simulink model "Simulation"  (R2019b)
settings: Solver=ode1  StartTime=0.0  StopTime=50  FixedStep=0.002  RelTol=1e-3  EnableMultiTasking=on
values from neighbouring files (symbols this model uses):
  Co = 0.1285    [Setup_sim.m]
  Dp = 0.024*0    (= 0)    [Setup_sim.m]
  Dr = 0.0690    (= 0.069)    [Setup_sim.m]
  g = 0.981    [Setup_sim.m]
  init_condi = pi/180*[5, 5, 0, 0]    [Setup_sim.m]
  Jp = 0.0012    [Setup_sim.m]    (also in parameters.mat)
  Jr = 0.0083    [Setup_sim.m]    (also in parameters.mat = 0.0038)
  K_AMP = 1    [Setup_sim.m]
  K_CT = lqr(Ai,Bi,Qx,Qu)    [Setup_sim.m]
  Lp = 0.3111    [Setup_sim.m]    (also in parameters.mat = 0.337)
  Lr = 0.1270    (= 0.127)    [Setup_sim.m]    (also in parameters.mat)
  Mp = 0.1270    (= 0.127)    [Setup_sim.m]
  sysc = ss(A,B,C,D)    [Setup_sim.m]
  VMAX_DAC = 10    [Setup_sim.m]
undefined symbols (not defined in the file or in its folder): DiscIntNeverNeededParam, L_CT, VMAX_AMP
libraries: simulink_extras x7
settings Model: ExtModeTrigDuration=10000  Creator=MLevis  LastModifiedBy=albin
settings SolverCC: PositivePriorityOrder=on
settings DataIOCC: LimitDataPoints=on  SaveFormat=Array  SignalLoggingSaveFormat=ModelDataLogs  ReturnWorkspaceOutputs=off
settings OptimizationCC: BooleanDataType=off  OptimizeBlockIOStorage=off  BufferReuse=off  GlobalBufferReuse=off  ExpressionFolding=off  ExpressionDepthLimit=2147483647  LocalBlockOutputs=off  InitFltsAndDblsToZero=on  LifeSpan=inf  OptimizeDataStoreBuffers=off  BusAssignmentInplaceUpdate=off
settings DebuggingCC: SaveWithParameterizedLinksMsg=none  UnderspecifiedInitializationDetection=Classic  MergeDetectMultiDrivingBlocksExec=none  SignalResolutionControl=TryResolveAllWithWarning  MultiTaskDSMMsg=warning  MultiTaskCondExecSysMsg=none  FcnCallInpInsideContextMsg=warning  StateNameClashWarn=warning  SFUnexpectedBacktrackingDiag=warning  SFNoUnconditionalDefaultTransitionDiag=warning  ArithmeticOperatorsInVariantConditions=warning
settings HardwareCC: ProdBitPerPointer=32  ProdBitPerSizeT=32  ProdBitPerPtrDiffT=32  ProdLargestAtomicFloat=None  ProdIntDivRoundTo=Undefined  ProdEndianess=Unspecified  ProdWordSize=32  ProdHWDeviceType=32-bit Generic  TargetHWDeviceType=32-bit Generic
settings ModelReferenceCC: PropagateSignalLabelsOutOfModel=off
settings SFSimCC: SimUseLocalCustomCode=off  CustomCodeUndefinedFunction=UseInterfaceOnly
settings RTWCC: Description=Quarc Win32 Target  SystemTargetFile=quarc_windows.tlc  TemplateMakefile=quarc_default_tmf  RTWUseLocalCustomCode=off
settings CodeAppCC: StateflowObjectComments=on
settings STFCustomTargetCC: TargetFcnLib=ansi_tfl_tmw.mat  TargetPreCompLibLocation=C:\PROGRA~3\QUARC\lib\2015a\windows\release  GeneratePreprocessorConditionals=Disable all  CPPClassGenCompliant=on  GRTInterface=on  SystemTargetFile=quarc_windows.tlc
settings GRTTargetCC: TargetFcnLib=ansi_tfl_tmw.mat  TargetPreCompLibLocation=C:\PROGRA~3\QUARC\lib\2015a\windows\release  TargetLangStandard=C89/C90 (ANSI)  ParMdlRefBuildCompliant=off  CompOptLevelCompliant=off  ConcurrentExecutionCompliant=off  GeneratePreprocessorConditionals=Disable all  CombineOutputUpdateFcns=off  MatFileLogging=off  GRTInterface=on  UseToolchainInfoCompliant=off  ExtMode=on  ExtModeMexFile=quarc_comm
settings ConfigComp: CovMetricSettings=dw  CovHtmlReporting=on  CovSaveCumulativeToWorkspaceVar=on  CovSaveSingleToWorkspaceVar=on  CovExternalEMLEnable=off

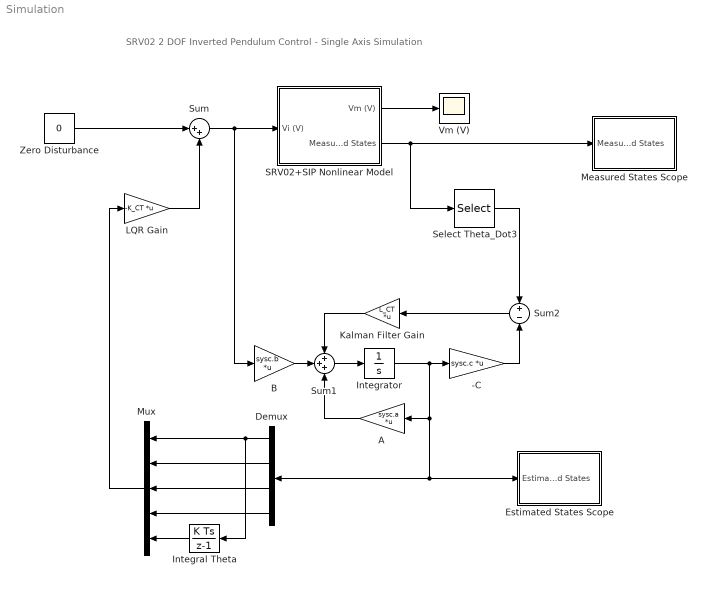
== system Simulation ==
  note: SRV02 2 DOF Inverted Pendulum Control - Single Axis Simulation
  -C : Gain  Gain=sysc.c  Multiplication=Matrix(K*u)
  A : Gain  Gain=sysc.a  Multiplication=Matrix(K*u)
  B : Gain  Gain=sysc.b  Multiplication=Matrix(K*u)
  Demux : Demux
  Estimated States Scope : Subsystem
  Integral Theta : DiscreteIntegrator  SampleTime=0.002  ICPrevOutput=DiscIntNeverNeededParam  ICPrevScaledInput=DiscIntNeverNeededParam
  Integrator : Integrator
  Kalman Filter Gain : Gain  Gain=L_CT  Multiplication=Matrix(K*u)
  LQR Gain : Gain  Gain=-K_CT  Multiplication=Matrix(K*u)  SaturateOnIntegerOverflow=on  OutDataTypeStr=Inherit: Same as input  ParamDataTypeStr=Inherit: Same as input
  Measured States Scope : Subsystem
  Mux : Mux  Inputs=5
  SRV02+SIP Nonlinear Model : Subsystem
  Select Theta_Dot3 : Selector  InputPortWidth=3  IndexOptions=Index vector (dialog)  Indices=[1 2]  OutputSizes=1
  Sum : Sum  Inputs=|++
  Sum1 : Sum  Inputs=+++
  Sum2 : Sum  Inputs=+|-
  Vm (V) : Scope
  Zero Disturbance : Constant  Value=0
  wires:
  LQR Gain/1 -> Sum/2
  B/1 -> Sum1/2
  Sum1/1 -> Integrator/1
  Integrator/1 -> Demux/1, Estimated States Scope/1(Estimated States), A/1, -C/1
  -C/1 -> Sum2/2
  Sum2/1 -> Kalman Filter Gain/1
  Kalman Filter Gain/1 -> Sum1/1
  A/1 -> Sum1/3
  Sum/1 -> SRV02+SIP Nonlinear Model/1(Vi (V)), B/1
  SRV02+SIP Nonlinear Model/2(Measured States) -> Measured States Scope/1(Measured States), Select Theta_Dot3/1
  SRV02+SIP Nonlinear Model/1(Vm (V)) -> Vm (V)/1
  Zero Disturbance/1 -> Sum/1
  Select Theta_Dot3/1 -> Sum2/1
  Demux/1 -> Integral Theta/1, Mux/1
  Demux/2 -> Mux/2
  Demux/3 -> Mux/3
  Demux/4 -> Mux/4
  Mux/1 -> LQR Gain/1
  Integral Theta/1 -> Mux/5

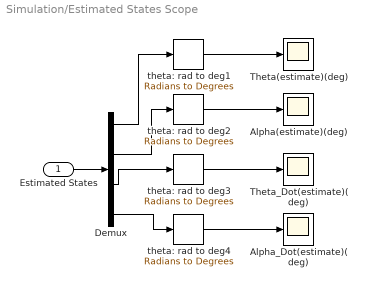
== system Simulation/Estimated States Scope ==
  Estimated States : Inport
  Alpha(estimate)(deg) : Scope
  Alpha_Dot(estimate)(deg) : Scope
  Demux : Demux
  Theta(estimate)(deg) : Scope
  Theta_Dot(estimate)(deg) : Scope
  theta: rad to deg{1..4} (4 alike) : simulink_extras/Transformations/Radians to Degrees
  wires:
  Demux/1 -> theta: rad to deg1/1
  theta: rad to deg1/1 -> Theta(estimate)(deg)/1
  theta: rad to deg2/1 -> Alpha(estimate)(deg)/1
  Demux/2 -> theta: rad to deg2/1
  theta: rad to deg3/1 -> Theta_Dot(estimate)(deg)/1
  Demux/3 -> theta: rad to deg3/1
  theta: rad to deg4/1 -> Alpha_Dot(estimate)(deg)/1
  Demux/4 -> theta: rad to deg4/1
  Estimated States/1 -> Demux/1

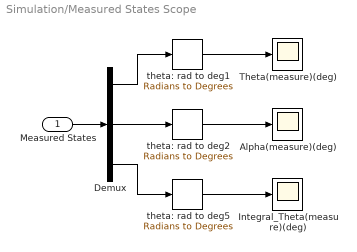
== system Simulation/Measured States Scope ==
  Measured States : Inport
  Alpha(measure)(deg) : Scope
  Demux : Demux  Outputs=3
  Integral_Theta(measure)(deg) : Scope
  Theta(measure)(deg) : Scope
  theta: rad to deg1 : simulink_extras/Transformations/Radians to Degrees
  theta: rad to deg2 : simulink_extras/Transformations/Radians to Degrees
  theta: rad to deg5 : simulink_extras/Transformations/Radians to Degrees
  wires:
  Measured States/1 -> Demux/1
  theta: rad to deg5/1 -> Integral_Theta(measure)(deg)/1
  theta: rad to deg2/1 -> Alpha(measure)(deg)/1
  theta: rad to deg1/1 -> Theta(measure)(deg)/1
  Demux/1 -> theta: rad to deg1/1
  Demux/2 -> theta: rad to deg2/1
  Demux/3 -> theta: rad to deg5/1

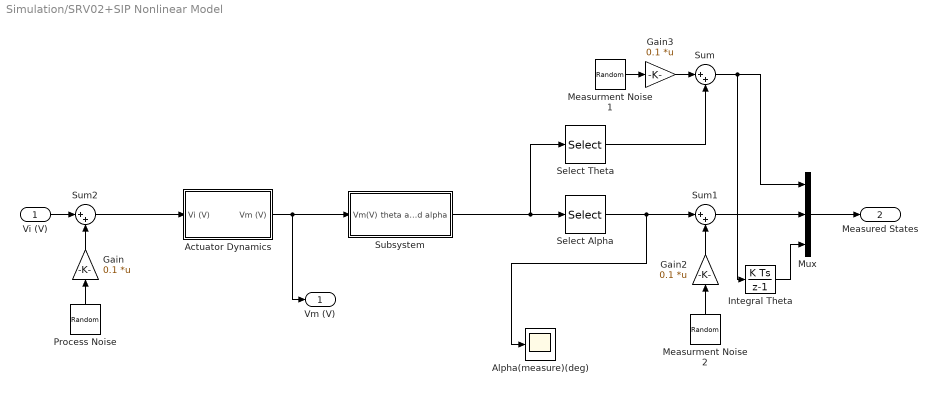
== system Simulation/SRV02+SIP Nonlinear Model ==
  Vi (V) : Inport
  Actuator Dynamics : Subsystem
  Alpha(measure)(deg) : Scope
  Gain : Gain  Gain=0.1  Multiplication=Matrix(K*u)  SaturateOnIntegerOverflow=on  OutDataTypeStr=Inherit: Same as input  ParamDataTypeStr=Inherit: Same as input
  Gain2 : Gain  Gain=0.1  Multiplication=Matrix(K*u)  SaturateOnIntegerOverflow=on  OutDataTypeStr=Inherit: Same as input  ParamDataTypeStr=Inherit: Same as input
  Gain3 : Gain  Gain=0.1  Multiplication=Matrix(K*u)  SaturateOnIntegerOverflow=on  OutDataTypeStr=Inherit: Same as input  ParamDataTypeStr=Inherit: Same as input
  Integral Theta : DiscreteIntegrator  SampleTime=0.002  ICPrevOutput=DiscIntNeverNeededParam  ICPrevScaledInput=DiscIntNeverNeededParam
  Measurment Noise 1 : RandomNumber  Variance=0.01
  Measurment Noise 2 : RandomNumber  Variance=0.01
  Mux : Mux  Inputs=3
  Process Noise : RandomNumber  Variance=50
  Select Alpha : Selector  InputPortWidth=2  IndexOptions=Index vector (dialog)  Indices=2  OutputSizes=1
  Select Theta : Selector  InputPortWidth=2  IndexOptions=Index vector (dialog)  Indices=1  OutputSizes=1
  Subsystem : Subsystem
  Sum : Sum  Inputs=|++
  Sum1 : Sum  Inputs=|++
  Sum2 : Sum  Inputs=|++
  Vm (V) : Outport  VectorParamsAs1DForOutWhenUnconnected=off
  Measured States : Outport  Port=2  VectorParamsAs1DForOutWhenUnconnected=off
  wires:
  Actuator Dynamics/1(Vm (V)) -> Subsystem/1(Vm(V)), Vm (V)/1
  Mux/1 -> Measured States/1
  Integral Theta/1 -> Mux/3
  Select Alpha/1 -> Sum1/1, Alpha(measure)(deg)/1
  Subsystem/1(theta and alpha) -> Select Alpha/1, Select Theta/1
  Select Theta/1 -> Sum/2
  Sum/1 -> Integral Theta/1, Mux/1
  Sum1/1 -> Mux/2
  Sum2/1 -> Actuator Dynamics/1(Vi (V))
  Vi (V)/1 -> Sum2/1
  Process Noise/1 -> Gain/1
  Gain/1 -> Sum2/2
  Measurment Noise 1/1 -> Gain3/1
  Gain3/1 -> Sum/1
  Gain2/1 -> Sum1/2
  Measurment Noise 2/1 -> Gain2/1

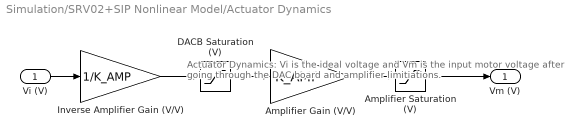
== system Simulation/SRV02+SIP Nonlinear Model/Actuator Dynamics ==
  note: Actuator Dynamics: Vi is the ideal voltage and Vm is the
      | input motor voltage after going through the DAC board and amplifier limitiations.
  Vi (V) : Inport
  Amplifier Gain (V/V) : Gain  Gain=K_AMP
  Amplifier Saturation (V) : Saturate  UpperLimit=VMAX_AMP  LowerLimit=-VMAX_AMP
  DACB Saturation (V) : Saturate  UpperLimit=VMAX_DAC  LowerLimit=-VMAX_DAC
  Inverse Amplifier Gain (V/V) : Gain  Gain=1/K_AMP
  Vm (V) : Outport  VectorParamsAs1DForOutWhenUnconnected=off
  wires:
  Inverse Amplifier Gain (V/V)/1 -> DACB Saturation (V)/1
  DACB Saturation (V)/1 -> Amplifier Gain (V/V)/1
  Amplifier Gain (V/V)/1 -> Amplifier Saturation (V)/1
  Vi (V)/1 -> Inverse Amplifier Gain (V/V)/1
  Amplifier Saturation (V)/1 -> Vm (V)/1

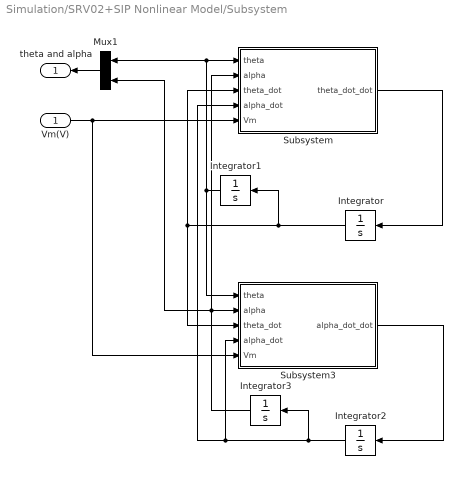
== system Simulation/SRV02+SIP Nonlinear Model/Subsystem ==
  Vm(V) : Inport
  Integrator : Integrator  InitialCondition=init_condi(3)
  Integrator1 : Integrator  InitialCondition=init_condi(1)
  Integrator2 : Integrator  InitialCondition=init_condi(4)
  Integrator3 : Integrator  InitialCondition=init_condi(2)
  Mux1 : Mux  Inputs=2
  Subsystem : Subsystem
  Subsystem3 : Subsystem
  theta and alpha : Outport  VectorParamsAs1DForOutWhenUnconnected=off
  wires:
  Mux1/1 -> theta and alpha/1
  Integrator3/1 -> Subsystem/2(alpha), Subsystem3/2(alpha), Mux1/2
  Integrator2/1 -> Subsystem3/4(alpha_dot), Subsystem/4(alpha_dot), Integrator3/1
  Subsystem3/1(alpha_dot_dot) -> Integrator2/1
  Integrator1/1 -> Subsystem/1(theta), Mux1/1, Subsystem3/1(theta)
  Integrator/1 -> Subsystem/3(theta_dot), Subsystem3/3(theta_dot), Integrator1/1
  Subsystem/1(theta_dot_dot) -> Integrator/1
  Vm(V)/1 -> Subsystem3/5(Vm), Subsystem/5(Vm)

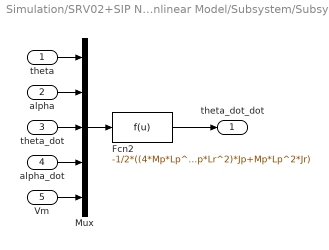
== system Simulation/SRV02+SIP Nonlinear Model/Subsystem/Subsystem ==
  theta : Inport
  alpha : Inport  Port=2
  theta_dot : Inport  Port=3
  alpha_dot : Inport  Port=4
  Vm : Inport  Port=5
  Fcn2 : Fcn  Expr=-1/2*((4*Mp*Lp^2*u(2)*u(1)*u(4)-8*Co*u(5)+8*Dr*u(3))*Jp+(Mp^2*Lp^4*u(2)*u(3)+4*Mp*Lp*Lr*Dp)*u(4))/((4*Jr+4*Mp*Lr^2)*Jp+Mp*Lp^2*Jr)-(-1/2)*((Mp^2*Lp^3*Lr*u(3)^2+20*Mp^2*Lp^2*Lr*g)*u(2)-2*Mp*Lp^2*Dr*u(3)+2*Mp*Lp^2*Co*u(5))/((4*Jr+4*Mp*Lr^2)*Jp+Mp*Lp^2*Jr)
  Mux : Mux  Inputs=5
  theta_dot_dot : Outport  VectorParamsAs1DForOutWhenUnconnected=off
  wires:
  Fcn2/1 -> theta_dot_dot/1
  Vm/1 -> Mux/5
  alpha_dot/1 -> Mux/4
  theta_dot/1 -> Mux/3
  alpha/1 -> Mux/2
  theta/1 -> Mux/1
  Mux/1 -> Fcn2/1

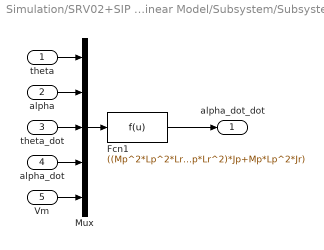
== system Simulation/SRV02+SIP Nonlinear Model/Subsystem/Subsystem3 ==
  theta : Inport
  alpha : Inport  Port=2
  theta_dot : Inport  Port=3
  alpha_dot : Inport  Port=4
  Vm : Inport  Port=5
  Fcn1 : Fcn  Expr=((Mp^2*Lp^2*Lr^2+Mp*Lp^2*Jr)*u(3)^2+20*Jr*Mp*Lp*g+20*Mp^2*Lr^2*Lp*g)*u(2)/((4*Jr+4*Mp*Lr^2)*Jp+Mp*Lp^2*Jr)+(2*Mp*Lr*Lp*Co*u(5)-2*Mp*Lr*Lp*Dr*u(3)-(Mp^2*Lp^3*Lr*u(2)*u(3)+4*Jr*Dp+4*Mp*Lr^2*Dp)*u(4))/((4*Jr+4*Mp*Lr^2)*Jp+Mp*Lp^2*Jr)
  Mux : Mux  Inputs=5
  alpha_dot_dot : Outport  VectorParamsAs1DForOutWhenUnconnected=off
  wires:
  Fcn1/1 -> alpha_dot_dot/1
  Vm/1 -> Mux/5
  alpha_dot/1 -> Mux/4
  theta_dot/1 -> Mux/3
  alpha/1 -> Mux/2
  theta/1 -> Mux/1
  Mux/1 -> Fcn1/1
